simulink model "vector_projection_to_plane"  (Simulink 6.2)
settings: Solver=ode45  StartTime=0.0  StopTime=10.0  RelTol=1e-3
undefined symbols (not defined in the file): vector_projection_onto_plane
settings Model: LastModifiedBy=Mads
settings DebuggingCC: SolverPrmCheckMsg=warning

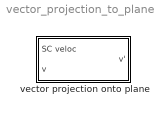
== system vector_projection_to_plane ==
  vector projection onto plane : Subsystem

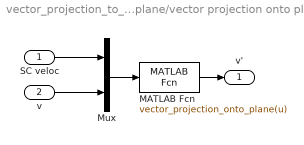
== system vector_projection_to_plane/vector projection onto plane ==
  SC veloc : Inport  Port=1  LatchInput=off
  v : Inport  Port=2  LatchInput=off
  MATLAB Fcn : MATLABFcn  MATLABFcn=vector_projection_onto_plane(u)
  Mux : Mux  Inputs=2
  v' : Outport
  wires:
  SC veloc/1 -> Mux/1
  MATLAB Fcn/1 -> v'/1
  v/1 -> Mux/2
  Mux/1 -> MATLAB Fcn/1
